simulink model "A_ASK_ruido"  (Simulink 8.3)
settings: Solver=VariableStepDiscrete  StartTime=0.0  StopTime=sim_t  RelTol=1e-3
undefined symbols (not defined in the file): A1a, A2a, A3a, BSTa, PZa, STa
libraries: commrandsrc2 x1, dsparch4 x1
settings Model: Creator=usuario  LastModifiedBy=C.JO2COR
settings OptimizationCC: ExpressionDepthLimit=2147483647  InitFltsAndDblsToZero=on
settings DebuggingCC: SaveWithParameterizedLinksMsg=none  SignalResolutionControl=TryResolveAllWithWarning  MultiTaskDSMMsg=warning  MultiTaskCondExecSysMsg=none  FrameProcessingCompatibilityMsg=error
settings SFSimCC: SimParseCustomCode=off
settings GRTTargetCC: TargetFcnLib=ansi_tfl_tmw.mat
settings ConfigComp: CovMetricSettings=dw  CovHtmlReporting=on  CovSaveCumulativeToWorkspaceVar=on  CovSaveSingleToWorkspaceVar=on  CovExternalEMLEnable=off  CovSFcnEnable=off

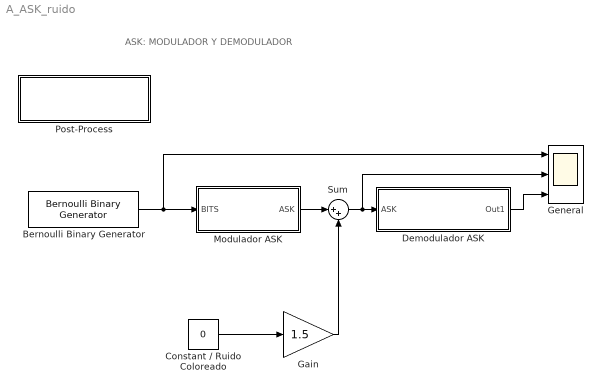
== system A_ASK_ruido ==
  note: ASK: MODULADOR Y DEMODULADOR
  Bernoulli Binary Generator : commrandsrc2/Bernoulli Binary Generator  P=PZa  seed=81  Ts=BSTa  frameBased=off  sampPerFrame=1  orient=off  outDataType=double
  Constant / Ruido Coloreado : Constant  Value=0
  Demodulador ASK : Subsystem
  Gain : Gain  Gain=1.5
  General : Scope  NumInputPorts=3
  Modulador ASK : Subsystem
  Post-Process : Subsystem  mask{sim_t=100, BSTa=5, FFa=5, A1a=8, A2a=0.5}
      mask prompts: sim_t "Sim Time [100]"; BSTa "Source Sample Time"; FFa "Freq. factor [1]"; A1a "Mod - Amp Sine 1 [2]"; A2a "Mod - Amp Sine 0 [.5]"
      mask init:
      | %sim_t = 100; %simulation time
      | %BST = 5; % source sample time
      | PZa = .4; % probability of zero
      | %ST = 1/20; % sample time
      | %SxP = 50; % samples per period
      | %A1 = 2; % amplitude sine 1 - mod.
      | %A2 = .5; % amplitude sine 2 - mod.
      | A3a = 1; % amplitude sine 3 - demod.
      | 
      | switch sim_t
      |     case 1
      |         sim_t = 50;
      |     case 2
      |         sim_t = 100;
      |     case 3
      |         sim_t = 250;
      |     case 4
      |         sim_t = 500;
      |     case 5
      |         sim_t = 1000;        
      | end
      | 
      | % Sample Time Source Configure
      | switch BSTa
      |     case 1
      |         BSTa = 5;
      |     case 2
      |         BSTa = 8;
      |     case 3
      |         BSTa = 10;
      |     case 4
      |         BSTa = 12;        
      | end
      | 
      | STa=(1/BSTa*1/4)*1/FFa;
      | %SxP=50*1/FF;
      | SxPa=(BSTa*10);
      | 
      | assignin('base','sim_t', sim_t );
      | assignin('base','FFa', FFa );
      | assignin('base','BSTa', BSTa );
      | assignin('base','PZa', PZa );
      | assignin('base','STa', STa );
      | assignin('base','SxPa', SxPa );
      | assignin('base','A1a', A1a );
      | assignin('base','A2a', A2a );
      | assignin('base','A3a', A3a );
      mask TypeOptions sim_t: 50 | 100 | 250 | 500 | 1000
      mask TypeOptions BSTa: 5 | 8 | 10 | 12
      mask Display: disp('Sim Parameters')
  Sum : Sum  Inputs=|++
  wires:
  Bernoulli Binary Generator/1 -> Modulador ASK/1(BITS), General/1
  Demodulador ASK/1(Out1) -> General/3
  Constant / Ruido Coloreado/1 -> Gain/1
  Modulador ASK/1(ASK) -> Sum/1
  Sum/1 -> General/2, Demodulador ASK/1(ASK)
  Gain/1 -> Sum/2

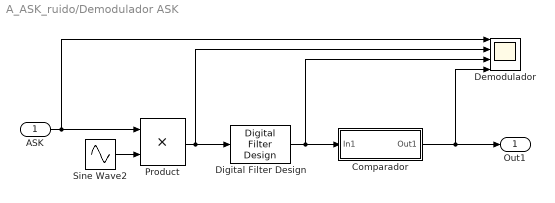
== system A_ASK_ruido/Demodulador ASK ==
  ASK : Inport
  Comparador : Subsystem
  Demodulador : Scope  NumInputPorts=4
  Digital Filter Design : dsparch4/Digital Filter Design  mwdsp_browser_bugfix_var=off
  Product : Product  RndMeth=Zero
  Sine Wave2 : Sin  SineType=Sample based  Amplitude=A3a  Frequency=2*10*pi  Samples=SxPa  SampleTime=STa
  Out1 : Outport
  wires:
  ASK/1 -> Product/1, Demodulador/1
  Sine Wave2/1 -> Product/2
  Product/1 -> Demodulador/2, Digital Filter Design/1
  Digital Filter Design/1 -> Demodulador/3, Comparador/1(In1)
  Comparador/1(Out1) -> Demodulador/4, Out1/1

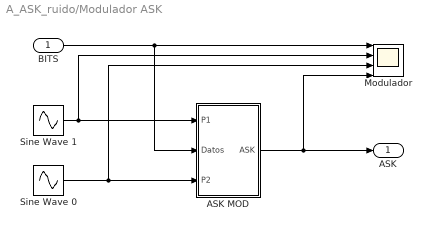
== system A_ASK_ruido/Modulador ASK ==
  BITS : Inport
  ASK MOD : Subsystem
  Modulador : Scope  NumInputPorts=4
  Sine Wave 0 : Sin  SineType=Sample based  Amplitude=A2a  Frequency=2*10*pi  Phase=-pi  Samples=SxPa  SampleTime=STa
  Sine Wave 1 : Sin  SineType=Sample based  Amplitude=A1a  Frequency=2*10*pi  Samples=SxPa  SampleTime=STa
  ASK : Outport
  wires:
  BITS/1 -> Modulador/1, ASK MOD/2(Datos)
  Sine Wave 1/1 -> ASK MOD/1(P1), Modulador/2
  Sine Wave 0/1 -> ASK MOD/3(P2), Modulador/3
  ASK MOD/1(ASK) -> Modulador/4, ASK/1

== system A_ASK_ruido/Post-Process ==

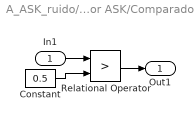
== system A_ASK_ruido/Demodulador ASK/Comparador ==
  In1 : Inport
  Constant : Constant  Value=0.5
  Relational Operator : RelationalOperator  Operator=>  OutDataTypeStr=boolean
  Out1 : Outport
  wires:
  Constant/1 -> Relational Operator/2
  In1/1 -> Relational Operator/1
  Relational Operator/1 -> Out1/1

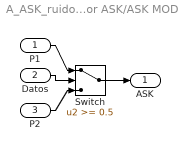
== system A_ASK_ruido/Modulador ASK/ASK MOD ==
  P1 : Inport
  Datos : Inport  Port=2
  P2 : Inport  Port=3
  Switch : Switch  Threshold=0.5
  ASK : Outport
  wires:
  P1/1 -> Switch/1
  Datos/1 -> Switch/2
  Switch/1 -> ASK/1
  P2/1 -> Switch/3
